simulink model "V_f_control_cinematico_PD"  (R2021b)
settings: Solver=VariableStepAuto  StartTime=0.0  StopTime=110  RelTol=1e-3
libraries: dsparch4 x6, slpidlib x3, simulink x2
settings Model: Creator=bmr  LastModifiedBy=bmr

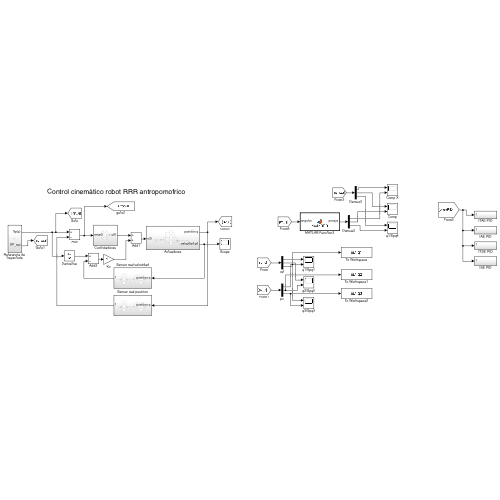
[thumbnail: Simulink's stored preview of the top-level diagram]
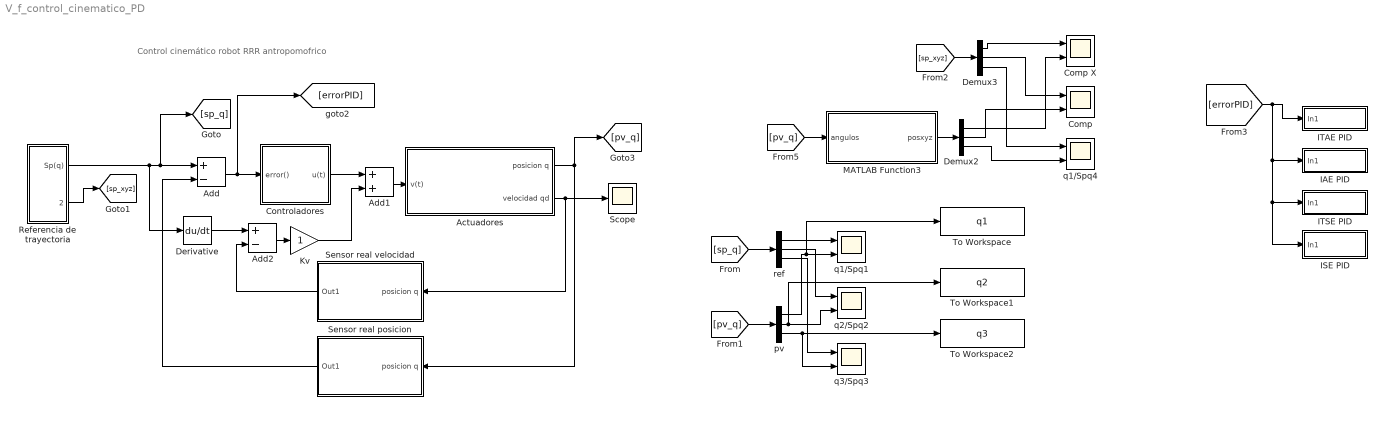
== system V_f_control_cinematico_PD ==
  note: Control cinemático robot RRR antropomofrico
  Actuadores : Subsystem
  Add : Sum  Inputs=+-
  Add1 : Sum
  Add2 : Sum  Inputs=+-
  Comp : Scope  NumInputPorts=2
  Comp X : Scope  NumInputPorts=2
  Controladores : Subsystem
  Demux2 : Demux  Outputs=3
  Demux3 : Demux  Outputs=3
  Derivative : Derivative
  IAE PID : Subsystem
  ISE PID : Subsystem
  ITAE PID : Subsystem
  ITSE PID : Subsystem
  Kv : Gain
  MATLAB Function3 : MATLAB Function  TreatAsAtomicUnit=on
  Referencia de trayectoria : Subsystem
  Scope : Scope
  Sensor real posicion : Subsystem
  Sensor real velocidad : Subsystem
  To Workspace : ToWorkspace  VariableName=q1  SampleTime=0.1
  To Workspace1 : ToWorkspace  VariableName=q2  SampleTime=0.1
  To Workspace2 : ToWorkspace  VariableName=q3  SampleTime=0.1
  pv : Demux  Outputs=3
  q1/Spq1 : Scope  NumInputPorts=2
  q1/Spq4 : Scope  NumInputPorts=2
  q2/Spq2 : Scope  NumInputPorts=2
  q3/Spq3 : Scope  NumInputPorts=2
  ref : Demux  Outputs=3
  wires:
  Add/1 -> [errorPID], Controladores/1(error())
  Actuadores/1(posicion q) -> Sensor real posicion/1(posicion q), [pv_q]
  Actuadores/2(velocidad qd) -> Sensor real velocidad/1(posicion q), Scope/1
  Sensor real posicion/1(Out1) -> Add/2
  [pv_q] -> MATLAB Function3/1(angulos)
  MATLAB Function3/1(posxyz) -> Demux2/1
  Demux2/1 -> Comp X/2
  Demux2/2 -> Comp/2
  Demux2/3 -> q1/Spq4/2
  Referencia de trayectoria/2(SP_xyz) -> [sp_xyz]
  [sp_xyz] -> Demux3/1
  Demux3/1 -> Comp X/1
  Demux3/2 -> Comp/1
  Demux3/3 -> q1/Spq4/1
  Sensor real velocidad/1(Out1) -> Add2/2
  Controladores/1(u(t)) -> Add1/1
  Add1/1 -> Actuadores/1(v(t))
  Derivative/1 -> Add2/1
  Add2/1 -> Kv/1
  Kv/1 -> Add1/2
  ref/1 -> q1/Spq1/1
  pv/1 -> To Workspace/1, q1/Spq1/2
  [pv_q] -> pv/1
  [sp_q] -> ref/1
  ref/2 -> q2/Spq2/1
  pv/2 -> q2/Spq2/2, To Workspace1/1
  pv/3 -> q3/Spq3/2, To Workspace2/1
  ref/3 -> q3/Spq3/1
  [errorPID] -> ISE PID/1(In1), ITSE PID/1(In1), IAE PID/1(In1), ITAE PID/1(In1)
  Referencia de trayectoria/1(Sp(q)) -> [sp_q], Add/1, Derivative/1

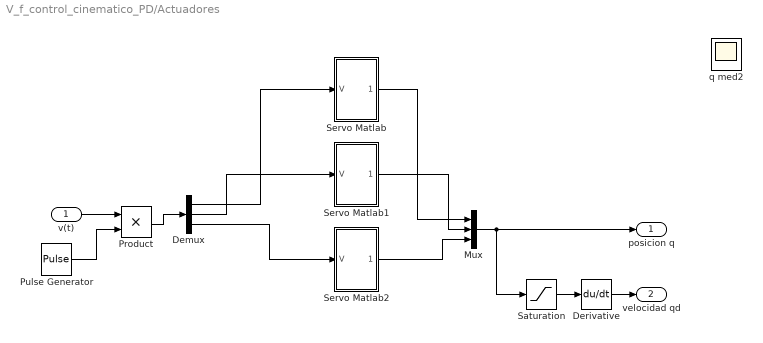
== system V_f_control_cinematico_PD/Actuadores ==
  v(t) : Inport
  Demux : Demux  Outputs=3
  Derivative : Derivative
  Mux : Mux  Inputs=3
  Product : Product
  Pulse Generator : DiscretePulseGenerator  PulseType=Time based  Period=0.001  PulseWidth=50
  Saturation : Saturate  UpperLimit=pi  LowerLimit=-pi
  Servo Matlab : Subsystem
  Servo Matlab1 : Subsystem
  Servo Matlab2 : Subsystem
  q med2 : Scope
  posicion q : Outport
  velocidad qd : Outport  Port=2
  wires:
  Mux/1 -> posicion q/1, Saturation/1
  Derivative/1 -> velocidad qd/1
  Demux/1 -> Servo Matlab/1(V)
  Demux/2 -> Servo Matlab1/1(V)
  Demux/3 -> Servo Matlab2/1(V)
  Servo Matlab2/1(Out1) -> Mux/3
  Servo Matlab1/1(Out1) -> Mux/2
  Servo Matlab/1(Out1) -> Mux/1
  Pulse Generator/1 -> Product/2
  v(t)/1 -> Product/1
  Product/1 -> Demux/1
  Saturation/1 -> Derivative/1

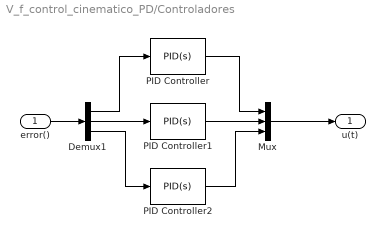
== system V_f_control_cinematico_PD/Controladores ==
  error() : Inport
  Demux1 : Demux  Outputs=3
  Mux : Mux  Inputs=3
  PID Controller : slpidlib/PID Controller  Controller=PID  Form=Parallel  TimeDomain=Continuous-time  UseExternalTs=off  SampleTime=-1  IntegratorMethod=Forward Euler  FilterMethod=Forward Euler  ControllerParametersSource=internal  P=382.208361491745  I=6.52154880893142  D=-1.71522518850909  UseFilter=on  N=222.832759250678  TunerSelectOption=Transfer Function Based (PID Tuner App)  InitialConditionSource=internal  InitialConditionForIntegrator=0  InitialConditionForFilter=0  DifferentiatorICPrevScaledInput=0  ExternalReset=none  TrackingMode=off  Kt=1  LimitOutput=on  SatLimitsSource=internal  UpperSaturationLimit=32000  LowerSaturationLimit=-32000  LinearizeAsGain=on  AntiWindupMode=none  Kb=1  POutMin=[]  POutMax=[]  IOutMin=[]  IOutMax=[]  DOutMin=[]  DOutMax=[]  NOutMin=[]  NOutMax=[]  SumOutMin=[]  SumOutMax=[]  SaturationOutMin=[]  SaturationOutMax=[]  PParamMin=[]  PParamMax=[]  IParamMin=[]  IParamMax=[]  DParamMin=[]  DParamMax=[]  NParamMin=[]  NParamMax=[]  KbParamMin=[]  KbParamMax=[]  KtParamMin=[]  KtParamMax=[]  KbOutMin=[]  KbOutMax=[]  KtOutMin=[]  KtOutMax=[]  IntegratorOutMin=[]  IntegratorOutMax=[]  FilterOutMin=[]  FilterOutMax=[]  SumI1OutMin=[]  SumI1OutMax=[]  SumI2OutMin=[]  SumI2OutMax=[]  SumI3OutMin=[]  SumI3OutMax=[]  SumI4OutMin=[]  SumI4OutMax=[]  SumDOutMin=[]  SumDOutMax=[]  DifferentiatorOutMin=[]  DifferentiatorOutMax=[]  FilterDiffOutCoefMin=[]  FilterDiffOutCoefMax=[]  ReciprocalOutMin=[]  ReciprocalOutMax=[]  SumDenOutMin=[]  SumDenOutMax=[]  SumNumOutMin=[]  SumNumOutMax=[]  DivideOutMin=[]  DivideOutMax=[]  UdiffTsProdOutMin=[]  UdiffTsProdOutMax=[]  NTsProdOutMin=[]  NTsProdOutMax=[]  UintegralTsProdOutMin=[]  UintegralTsProdOutMax=[]  UngainTsProdOutMin=[]  UngainTsProdOutMax=[]  IntegratorContinuousStateAttributes=''  IntegratorStateMustResolveToSignalObject=off  IntegratorRTWStateStorageClass=Auto  FilterContinuousStateAttributes=''  FilterStateMustResolveToSignalObject=off  FilterRTWStateStorageClass=Auto  ParallelPVariant=InternalParameters  IdealPVariant=Disabled  IVariant=InternalParameters  DVariant=InternalParameters  IntegratorVariant=Continuous  SatVariant=Enabled  AWVariant=Passthrough  PCopyVariant=Disabled  TRVariant=Disabled  FdbkBlocksVariant=Forward  IdealPFdbkVariant=Disabled  SatFdbkVariant=Disabled  DerivativeFilterVariant=ContFilter  NVariant=InternalParameters  NCopyVariant=Disabled  FilterICVariant=InternalICsFilter  IntegratorICVariant=InternalICs  ExternalResetVariant=Disabled  TRSumVariant=Passthrough  SumFdbkVariant=Disabled  SumVariant=Sum_PID  TsampFilterVariant=InternalTs  TsampNgainVariant=Passthrough  TsampIntegralVariant=Passthrough  ExternalSaturationOutDataTypeStr=Inherit: Same as second input
  PID Controller1 : slpidlib/PID Controller  Controller=PID  Form=Parallel  TimeDomain=Continuous-time  UseExternalTs=off  SampleTime=-1  IntegratorMethod=Forward Euler  FilterMethod=Forward Euler  ControllerParametersSource=internal  P=380.744284661777  I=6.49105516326343  D=17.2266060618832  UseFilter=on  N=222.832759250678  TunerSelectOption=Transfer Function Based (PID Tuner App)  InitialConditionSource=internal  InitialConditionForIntegrator=0  InitialConditionForFilter=0  DifferentiatorICPrevScaledInput=0  ExternalReset=none  TrackingMode=off  Kt=1  LimitOutput=on  SatLimitsSource=internal  UpperSaturationLimit=32000  LowerSaturationLimit=-32000  LinearizeAsGain=on  AntiWindupMode=none  Kb=1  POutMin=[]  POutMax=[]  IOutMin=[]  IOutMax=[]  DOutMin=[]  DOutMax=[]  NOutMin=[]  NOutMax=[]  SumOutMin=[]  SumOutMax=[]  SaturationOutMin=[]  SaturationOutMax=[]  PParamMin=[]  PParamMax=[]  IParamMin=[]  IParamMax=[]  DParamMin=[]  DParamMax=[]  NParamMin=[]  NParamMax=[]  KbParamMin=[]  KbParamMax=[]  KtParamMin=[]  KtParamMax=[]  KbOutMin=[]  KbOutMax=[]  KtOutMin=[]  KtOutMax=[]  IntegratorOutMin=[]  IntegratorOutMax=[]  FilterOutMin=[]  FilterOutMax=[]  SumI1OutMin=[]  SumI1OutMax=[]  SumI2OutMin=[]  SumI2OutMax=[]  SumI3OutMin=[]  SumI3OutMax=[]  SumI4OutMin=[]  SumI4OutMax=[]  SumDOutMin=[]  SumDOutMax=[]  DifferentiatorOutMin=[]  DifferentiatorOutMax=[]  FilterDiffOutCoefMin=[]  FilterDiffOutCoefMax=[]  ReciprocalOutMin=[]  ReciprocalOutMax=[]  SumDenOutMin=[]  SumDenOutMax=[]  SumNumOutMin=[]  SumNumOutMax=[]  DivideOutMin=[]  DivideOutMax=[]  UdiffTsProdOutMin=[]  UdiffTsProdOutMax=[]  NTsProdOutMin=[]  NTsProdOutMax=[]  UintegralTsProdOutMin=[]  UintegralTsProdOutMax=[]  UngainTsProdOutMin=[]  UngainTsProdOutMax=[]  IntegratorContinuousStateAttributes=''  IntegratorStateMustResolveToSignalObject=off  IntegratorRTWStateStorageClass=Auto  FilterContinuousStateAttributes=''  FilterStateMustResolveToSignalObject=off  FilterRTWStateStorageClass=Auto  ParallelPVariant=InternalParameters  IdealPVariant=Disabled  IVariant=InternalParameters  DVariant=InternalParameters  IntegratorVariant=Continuous  SatVariant=Enabled  AWVariant=Passthrough  PCopyVariant=Disabled  TRVariant=Disabled  FdbkBlocksVariant=Forward  IdealPFdbkVariant=Disabled  SatFdbkVariant=Disabled  DerivativeFilterVariant=ContFilter  NVariant=InternalParameters  NCopyVariant=Disabled  FilterICVariant=InternalICsFilter  IntegratorICVariant=InternalICs  ExternalResetVariant=Disabled  TRSumVariant=Passthrough  SumFdbkVariant=Disabled  SumVariant=Sum_PID  TsampFilterVariant=InternalTs  TsampNgainVariant=Passthrough  TsampIntegralVariant=Passthrough  ExternalSaturationOutDataTypeStr=Inherit: Same as second input
  PID Controller2 : slpidlib/PID Controller  Controller=PID  Form=Parallel  TimeDomain=Continuous-time  UseExternalTs=off  SampleTime=-1  IntegratorMethod=Forward Euler  FilterMethod=Forward Euler  ControllerParametersSource=internal  P=307.461622992245  I=4.77261436567613  D=47.3820560934873  UseFilter=on  N=1.77827193646515  TunerSelectOption=Transfer Function Based (PID Tuner App)  InitialConditionSource=internal  InitialConditionForIntegrator=0  InitialConditionForFilter=0  DifferentiatorICPrevScaledInput=0  ExternalReset=none  TrackingMode=off  Kt=1  LimitOutput=on  SatLimitsSource=internal  UpperSaturationLimit=32000  LowerSaturationLimit=-32000  LinearizeAsGain=on  AntiWindupMode=none  Kb=1  POutMin=[]  POutMax=[]  IOutMin=[]  IOutMax=[]  DOutMin=[]  DOutMax=[]  NOutMin=[]  NOutMax=[]  SumOutMin=[]  SumOutMax=[]  SaturationOutMin=[]  SaturationOutMax=[]  PParamMin=[]  PParamMax=[]  IParamMin=[]  IParamMax=[]  DParamMin=[]  DParamMax=[]  NParamMin=[]  NParamMax=[]  KbParamMin=[]  KbParamMax=[]  KtParamMin=[]  KtParamMax=[]  KbOutMin=[]  KbOutMax=[]  KtOutMin=[]  KtOutMax=[]  IntegratorOutMin=[]  IntegratorOutMax=[]  FilterOutMin=[]  FilterOutMax=[]  SumI1OutMin=[]  SumI1OutMax=[]  SumI2OutMin=[]  SumI2OutMax=[]  SumI3OutMin=[]  SumI3OutMax=[]  SumI4OutMin=[]  SumI4OutMax=[]  SumDOutMin=[]  SumDOutMax=[]  DifferentiatorOutMin=[]  DifferentiatorOutMax=[]  FilterDiffOutCoefMin=[]  FilterDiffOutCoefMax=[]  ReciprocalOutMin=[]  ReciprocalOutMax=[]  SumDenOutMin=[]  SumDenOutMax=[]  SumNumOutMin=[]  SumNumOutMax=[]  DivideOutMin=[]  DivideOutMax=[]  UdiffTsProdOutMin=[]  UdiffTsProdOutMax=[]  NTsProdOutMin=[]  NTsProdOutMax=[]  UintegralTsProdOutMin=[]  UintegralTsProdOutMax=[]  UngainTsProdOutMin=[]  UngainTsProdOutMax=[]  IntegratorContinuousStateAttributes=''  IntegratorStateMustResolveToSignalObject=off  IntegratorRTWStateStorageClass=Auto  FilterContinuousStateAttributes=''  FilterStateMustResolveToSignalObject=off  FilterRTWStateStorageClass=Auto  ParallelPVariant=InternalParameters  IdealPVariant=Disabled  IVariant=InternalParameters  DVariant=InternalParameters  IntegratorVariant=Continuous  SatVariant=Enabled  AWVariant=Passthrough  PCopyVariant=Disabled  TRVariant=Disabled  FdbkBlocksVariant=Forward  IdealPFdbkVariant=Disabled  SatFdbkVariant=Disabled  DerivativeFilterVariant=ContFilter  NVariant=InternalParameters  NCopyVariant=Disabled  FilterICVariant=InternalICsFilter  IntegratorICVariant=InternalICs  ExternalResetVariant=Disabled  TRSumVariant=Passthrough  SumFdbkVariant=Disabled  SumVariant=Sum_PID  TsampFilterVariant=InternalTs  TsampNgainVariant=Passthrough  TsampIntegralVariant=Passthrough  ExternalSaturationOutDataTypeStr=Inherit: Same as second input
  u(t) : Outport
  wires:
  error()/1 -> Demux1/1
  PID Controller2/1 -> Mux/3
  Demux1/1 -> PID Controller/1
  PID Controller1/1 -> Mux/2
  PID Controller/1 -> Mux/1
  Mux/1 -> u(t)/1
  Demux1/2 -> PID Controller1/1
  Demux1/3 -> PID Controller2/1

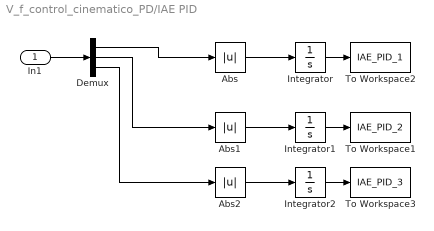
== system V_f_control_cinematico_PD/IAE PID ==
  In1 : Inport
  Abs : Abs
  Abs1 : Abs
  Abs2 : Abs
  Demux : Demux  Outputs=3
  Integrator : Integrator  LimitOutput=on  LowerSaturationLimit=0
  Integrator1 : Integrator  LimitOutput=on  LowerSaturationLimit=0
  Integrator2 : Integrator  LimitOutput=on  LowerSaturationLimit=0
  To Workspace1 : ToWorkspace  VariableName=IAE_PID_2  SampleTime=0.1
  To Workspace2 : ToWorkspace  VariableName=IAE_PID_1  SampleTime=0.1
  To Workspace3 : ToWorkspace  VariableName=IAE_PID_3  SampleTime=0.1
  wires:
  Abs/1 -> Integrator/1
  Integrator/1 -> To Workspace2/1
  Demux/2 -> Abs1/1
  Demux/1 -> Abs/1
  In1/1 -> Demux/1
  Abs1/1 -> Integrator1/1
  Integrator1/1 -> To Workspace1/1
  Integrator2/1 -> To Workspace3/1
  Abs2/1 -> Integrator2/1
  Demux/3 -> Abs2/1

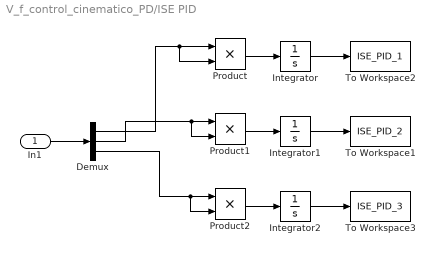
== system V_f_control_cinematico_PD/ISE PID ==
  In1 : Inport
  Demux : Demux  Outputs=3
  Integrator : Integrator  LimitOutput=on  LowerSaturationLimit=0
  Integrator1 : Integrator  LimitOutput=on  LowerSaturationLimit=0
  Integrator2 : Integrator  LimitOutput=on  LowerSaturationLimit=0
  Product : Product
  Product1 : Product
  Product2 : Product
  To Workspace1 : ToWorkspace  VariableName=ISE_PID_2  SampleTime=0.1
  To Workspace2 : ToWorkspace  VariableName=ISE_PID_1  SampleTime=0.1
  To Workspace3 : ToWorkspace  VariableName=ISE_PID_3  SampleTime=0.1
  wires:
  Product/1 -> Integrator/1
  Integrator/1 -> To Workspace2/1
  In1/1 -> Demux/1
  Integrator1/1 -> To Workspace1/1
  Product1/1 -> Integrator1/1
  Product2/1 -> Integrator2/1
  Integrator2/1 -> To Workspace3/1
  Demux/1 -> Product/2, Product/1
  Demux/2 -> Product1/2, Product1/1
  Demux/3 -> Product2/2, Product2/1

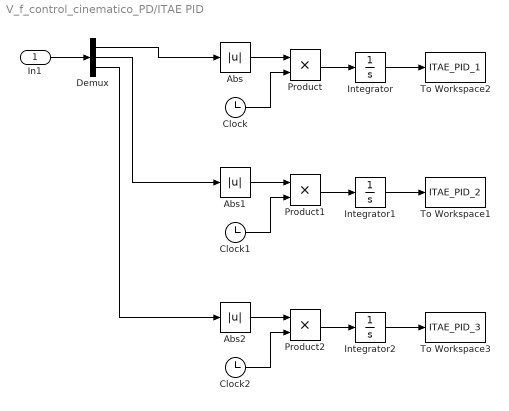
== system V_f_control_cinematico_PD/ITAE PID ==
  In1 : Inport
  Abs : Abs
  Abs1 : Abs
  Abs2 : Abs
  Clock : Clock
  Clock1 : Clock
  Clock2 : Clock
  Demux : Demux  Outputs=3
  Integrator : Integrator  LimitOutput=on  LowerSaturationLimit=0
  Integrator1 : Integrator  LimitOutput=on  LowerSaturationLimit=0
  Integrator2 : Integrator  LimitOutput=on  LowerSaturationLimit=0
  Product : Product
  Product1 : Product
  Product2 : Product
  To Workspace1 : ToWorkspace  VariableName=ITAE_PID_2  SampleTime=0.1
  To Workspace2 : ToWorkspace  VariableName=ITAE_PID_1  SampleTime=0.1
  To Workspace3 : ToWorkspace  VariableName=ITAE_PID_3  SampleTime=0.1
  wires:
  Clock/1 -> Product/2
  Abs/1 -> Product/1
  Integrator/1 -> To Workspace2/1
  Product/1 -> Integrator/1
  Clock1/1 -> Product1/2
  Product1/1 -> Integrator1/1
  Abs1/1 -> Product1/1
  Integrator1/1 -> To Workspace1/1
  Clock2/1 -> Product2/2
  Product2/1 -> Integrator2/1
  Abs2/1 -> Product2/1
  Integrator2/1 -> To Workspace3/1
  In1/1 -> Demux/1
  Demux/1 -> Abs/1
  Demux/2 -> Abs1/1
  Demux/3 -> Abs2/1

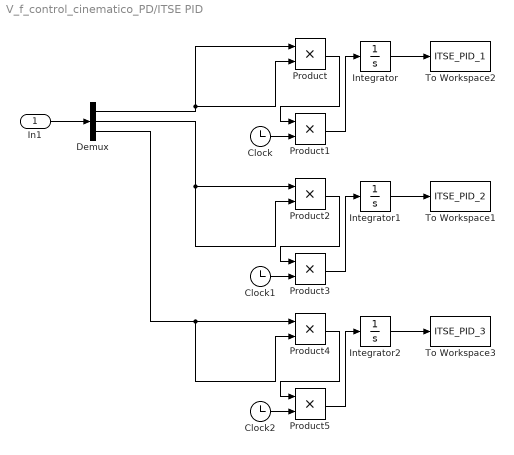
== system V_f_control_cinematico_PD/ITSE PID ==
  In1 : Inport
  Clock : Clock
  Clock1 : Clock
  Clock2 : Clock
  Demux : Demux  Outputs=3
  Integrator : Integrator  LimitOutput=on  LowerSaturationLimit=0
  Integrator1 : Integrator  LimitOutput=on  LowerSaturationLimit=0
  Integrator2 : Integrator  LimitOutput=on  LowerSaturationLimit=0
  Product{,1..5} (6 alike) : Product
  To Workspace1 : ToWorkspace  VariableName=ITSE_PID_2  SampleTime=0.1
  To Workspace2 : ToWorkspace  VariableName=ITSE_PID_1  SampleTime=0.1
  To Workspace3 : ToWorkspace  VariableName=ITSE_PID_3  SampleTime=0.1
  wires:
  Demux/1 -> Product/1, Product/2
  Integrator/1 -> To Workspace2/1
  Product/1 -> Product1/1
  Clock/1 -> Product1/2
  Product1/1 -> Integrator/1
  In1/1 -> Demux/1
  Integrator1/1 -> To Workspace1/1
  Product2/1 -> Product3/1
  Product3/1 -> Integrator1/1
  Demux/2 -> Product2/2, Product2/1
  Clock1/1 -> Product3/2
  Product4/1 -> Product5/1
  Product5/1 -> Integrator2/1
  Clock2/1 -> Product5/2
  Demux/3 -> Product4/2, Product4/1
  Integrator2/1 -> To Workspace3/1

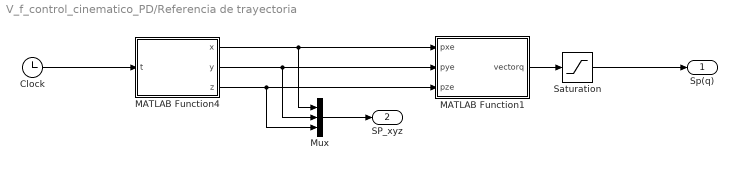
== system V_f_control_cinematico_PD/Referencia de trayectoria ==
  Clock : Clock
  MATLAB Function1 : MATLAB Function  TreatAsAtomicUnit=on
  MATLAB Function4 : MATLAB Function  TreatAsAtomicUnit=on
  Mux : Mux  Inputs=3
  Saturation : Saturate  UpperLimit=1.57  LowerLimit=-1.57
  Sp(q) : Outport
  SP_xyz : Outport  Port=2
  wires:
  MATLAB Function1/1(vectorq) -> Saturation/1
  Clock/1 -> MATLAB Function4/1(t)
  MATLAB Function4/3(z) -> Mux/3, MATLAB Function1/3(pze)
  MATLAB Function4/2(y) -> Mux/2, MATLAB Function1/2(pye)
  MATLAB Function4/1(x) -> Mux/1, MATLAB Function1/1(pxe)
  Saturation/1 -> Sp(q)/1
  Mux/1 -> SP_xyz/1

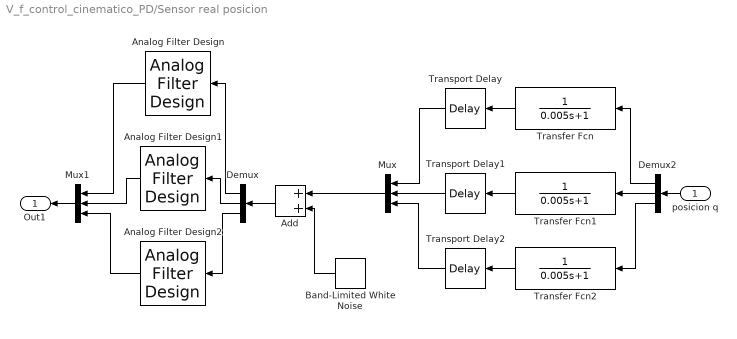
== system V_f_control_cinematico_PD/Sensor real posicion ==
  posicion q : Inport
  Add : Sum
  Analog Filter Design : dsparch4/Analog Filter Design  method=Butterworth  filttype=Lowpass  N=8  Wlo=30  Whi=80  Rp=2  Rs=40
  Analog Filter Design1 : dsparch4/Analog Filter Design  method=Butterworth  filttype=Lowpass  N=8  Wlo=30  Whi=80  Rp=2  Rs=40
  Analog Filter Design2 : dsparch4/Analog Filter Design  method=Butterworth  filttype=Lowpass  N=8  Wlo=30  Whi=80  Rp=2  Rs=40
  Band-Limited White Noise : simulink/Sources/Band-Limited White Noise  Cov=[0.001]  Ts=0.1  seed=[23341]
  Demux : Demux  Outputs=3
  Demux2 : Demux  Outputs=3
  Mux : Mux  Inputs=3
  Mux1 : Mux  Inputs=3
  Transfer Fcn : TransferFcn  Denominator=[0.005 1]
  Transfer Fcn1 : TransferFcn  Denominator=[0.005 1]
  Transfer Fcn2 : TransferFcn  Denominator=[0.005 1]
  Transport Delay : TransportDelay  DelayTime=0.05
  Transport Delay1 : TransportDelay  DelayTime=0.05
  Transport Delay2 : TransportDelay  DelayTime=0.05
  Out1 : Outport
  wires:
  Transfer Fcn1/1 -> Transport Delay1/1
  Demux2/3 -> Transfer Fcn2/1
  Transfer Fcn/1 -> Transport Delay/1
  Demux2/2 -> Transfer Fcn1/1
  Transport Delay/1 -> Mux/1
  Transfer Fcn2/1 -> Transport Delay2/1
  Transport Delay1/1 -> Mux/2
  Transport Delay2/1 -> Mux/3
  Demux2/1 -> Transfer Fcn/1
  posicion q/1 -> Demux2/1
  Band-Limited White Noise/1 -> Add/2
  Mux/1 -> Add/1
  Add/1 -> Demux/1
  Demux/1 -> Analog Filter Design/1
  Demux/2 -> Analog Filter Design1/1
  Demux/3 -> Analog Filter Design2/1
  Mux1/1 -> Out1/1
  Analog Filter Design/1 -> Mux1/1
  Analog Filter Design1/1 -> Mux1/2
  Analog Filter Design2/1 -> Mux1/3

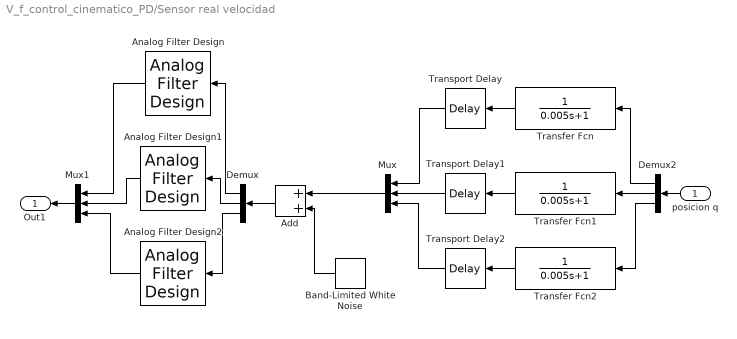
== system V_f_control_cinematico_PD/Sensor real velocidad ==
  posicion q : Inport
  Add : Sum
  Analog Filter Design : dsparch4/Analog Filter Design  method=Butterworth  filttype=Lowpass  N=8  Wlo=30  Whi=80  Rp=2  Rs=40
  Analog Filter Design1 : dsparch4/Analog Filter Design  method=Butterworth  filttype=Lowpass  N=8  Wlo=30  Whi=80  Rp=2  Rs=40
  Analog Filter Design2 : dsparch4/Analog Filter Design  method=Butterworth  filttype=Lowpass  N=8  Wlo=30  Whi=80  Rp=2  Rs=40
  Band-Limited White Noise : simulink/Sources/Band-Limited White Noise  Cov=[0.001]  Ts=0.1  seed=[23341]
  Demux : Demux  Outputs=3
  Demux2 : Demux  Outputs=3
  Mux : Mux  Inputs=3
  Mux1 : Mux  Inputs=3
  Transfer Fcn : TransferFcn  Denominator=[0.005 1]
  Transfer Fcn1 : TransferFcn  Denominator=[0.005 1]
  Transfer Fcn2 : TransferFcn  Denominator=[0.005 1]
  Transport Delay : TransportDelay  DelayTime=0.05
  Transport Delay1 : TransportDelay  DelayTime=0.05
  Transport Delay2 : TransportDelay  DelayTime=0.05
  Out1 : Outport
  wires:
  Transfer Fcn1/1 -> Transport Delay1/1
  Demux2/3 -> Transfer Fcn2/1
  Transfer Fcn/1 -> Transport Delay/1
  Demux2/2 -> Transfer Fcn1/1
  Transport Delay/1 -> Mux/1
  Transfer Fcn2/1 -> Transport Delay2/1
  Transport Delay1/1 -> Mux/2
  Transport Delay2/1 -> Mux/3
  Demux2/1 -> Transfer Fcn/1
  posicion q/1 -> Demux2/1
  Band-Limited White Noise/1 -> Add/2
  Mux/1 -> Add/1
  Add/1 -> Demux/1
  Demux/1 -> Analog Filter Design/1
  Demux/2 -> Analog Filter Design1/1
  Demux/3 -> Analog Filter Design2/1
  Mux1/1 -> Out1/1
  Analog Filter Design/1 -> Mux1/1
  Analog Filter Design1/1 -> Mux1/2
  Analog Filter Design2/1 -> Mux1/3

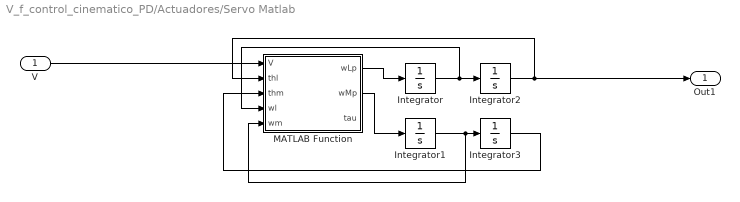
== system V_f_control_cinematico_PD/Actuadores/Servo Matlab ==
  V : Inport
  Integrator : Integrator  UpperSaturationLimit=pi/2  LowerSaturationLimit=-pi/2
  Integrator1 : Integrator
  Integrator2 : Integrator  LimitOutput=on  UpperSaturationLimit=pi/2  LowerSaturationLimit=-pi/2
  Integrator3 : Integrator  UpperSaturationLimit=pi/2  LowerSaturationLimit=-pi/2
  MATLAB Function : MATLAB Function  TreatAsAtomicUnit=on
  Out1 : Outport
  wires:
  V/1 -> MATLAB Function/1(V)
  Integrator2/1 -> Out1/1, MATLAB Function/2(thl)
  Integrator/1 -> Integrator2/1, MATLAB Function/4(wl)
  MATLAB Function/1(wLp) -> Integrator/1
  Integrator3/1 -> MATLAB Function/3(thm)
  MATLAB Function/2(wMp) -> Integrator1/1
  Integrator1/1 -> Integrator3/1, MATLAB Function/5(wm)

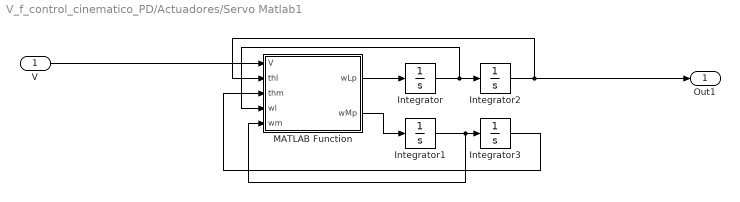
== system V_f_control_cinematico_PD/Actuadores/Servo Matlab1 ==
  V : Inport
  Integrator : Integrator  UpperSaturationLimit=pi/2  LowerSaturationLimit=-pi/2
  Integrator1 : Integrator
  Integrator2 : Integrator  InitialCondition=pi/2  LimitOutput=on  UpperSaturationLimit=pi/2  LowerSaturationLimit=-pi/2
  Integrator3 : Integrator  UpperSaturationLimit=pi/2  LowerSaturationLimit=-pi/2
  MATLAB Function : MATLAB Function  TreatAsAtomicUnit=on
  Out1 : Outport
  wires:
  V/1 -> MATLAB Function/1(V)
  Integrator2/1 -> Out1/1, MATLAB Function/2(thl)
  Integrator/1 -> Integrator2/1, MATLAB Function/4(wl)
  MATLAB Function/1(wLp) -> Integrator/1
  Integrator3/1 -> MATLAB Function/3(thm)
  MATLAB Function/2(wMp) -> Integrator1/1
  Integrator1/1 -> Integrator3/1, MATLAB Function/5(wm)

== system V_f_control_cinematico_PD/Actuadores/Servo Matlab2 ==
  V : Inport
  Integrator : Integrator  InitialCondition=-pi/2  UpperSaturationLimit=pi/2  LowerSaturationLimit=-pi/2
  Integrator1 : Integrator
  Integrator2 : Integrator  LimitOutput=on  UpperSaturationLimit=pi/2  LowerSaturationLimit=-pi/2
  Integrator3 : Integrator  UpperSaturationLimit=pi/2  LowerSaturationLimit=-pi/2
  MATLAB Function : MATLAB Function  TreatAsAtomicUnit=on
  Out1 : Outport
  wires:
  V/1 -> MATLAB Function/1(V)
  Integrator2/1 -> Out1/1, MATLAB Function/2(thl)
  Integrator/1 -> Integrator2/1, MATLAB Function/4(wl)
  MATLAB Function/1(wLp) -> Integrator/1
  Integrator3/1 -> MATLAB Function/3(thm)
  MATLAB Function/2(wMp) -> Integrator1/1
  Integrator1/1 -> Integrator3/1, MATLAB Function/5(wm)

== matlab function V_f_control_cinematico_PD/Actuadores/Servo Matlab/MATLAB Function ==
  data: V input; wLp output; thl input; thm input; wl input; wm input; wMp output; tau output
function [wLp,wMp,tau] = servomotor(V, thl,thm, wl, wm)
Kt = 1280.2;  % Torsional rigidity
Km = 10;      % Motor constant
Jm = 0.5;     % Motor inertia
Jl = 50*Jm;   % Load inertia
N = 20;       % Gear ratio
Bm = 0.1;     % Rotor viscous friction
Bl = 25;      % Load viscous friction
R = 20;       % Armature resistance
wLp = (-(Kt/Jl)*(thl - (thm/N))) - ((Bl*wl)/Jl);
wMp = (Km/Jm) * ((V - Km * wm)/R) - ((Bm * wm)/Jm) + (Kt/(N*Jm))*(thl - (thm/N));
%% https://www.mathworks.com/help/mpc/ug/servomechanism-controller.html?searchHighlight=mpc%20dc%20motor&s_tid=doc_srchtitle %%
% Torque maquina
tau = (Kt * thl) -((Kt/N)*thm);

== matlab function V_f_control_cinematico_PD/Referencia de trayectoria/MATLAB Function1 ==
  data: pxe input size=1; vectorq output size=3; pye input size=1; pze input size=1
function vectorq = cininvRRR(pxe,pye,pze)
%% Valores 
L1=0.2;L2=0.2;L3=0.2;
%% angulos
q1=atan2(pye,pxe);
cq3=(pxe^2 +pye^2 +pze^2 -L2^2 -L3^2)/(2*L2*L3);
%% Condicionante para la variable cq3
if (cq3>=1)
    cq3=1;
else
    cq3=0.001;
end 

q3=atan2(sqrt(1-cq3),cq3);
beta=atan2(pze,sqrt(pxe^2 +pye^2));
alfa=atan2(L3*sin(q3),L2 +L3*cq3);
q2=beta-alfa;
vectorq=[q1;q2;q3];

== matlab function V_f_control_cinematico_PD/MATLAB Function3 ==
  data: angulos input size=3; posxyz output size=3
%% Funcion cinematica directa
function posxyz = cindinRRR(angulos)
%% Vector angulo de 3 dim.
th1=angulos(1);
th2=angulos(2);
th3=angulos(3);
%% Valores eslabones
L1=0.2;L2=0.2;L3=0.2;
%% pos
xe=cos(th1)*(L3*cos(th2+th3) + L2*cos(th2));
ye=sin(th1)*(L3*cos(th2+th3) + L2*cos(th2));
ze=L1+(L3*sin(th2+th3)) +L2*sin(th2);
posxyz=[xe;ye;ze];

== matlab function V_f_control_cinematico_PD/Referencia de trayectoria/MATLAB Function4 ==
  data: x output; t input; y output; z output
function [x,y,z] = Trayectoria(t)

if (t>=0) && (t<15)
    x = 0.2;
    y = 0.0;
    z = 0.4;

elseif (t>=15) && (t<30) 
    x = 0.2;
    y = 0.0;
    z = 0.0;
elseif (t>=30) && (t<45)
    x = 0.0;
    y = 0.2;
    z = 0.0;

elseif (t>=45) && (t<60)
    x = 0.2;
    y = 0.0;
    z = 0.0;

elseif (t>=60) && (t<75)
    x = 0.0;
    y = -0.2;
    z = 0.0;


elseif (t>=75) && (t<90)
    x = 0.4;
    y = 0.0;
    z = 0.2;


elseif (t>=90) && (t<105)
    x = 0.0;
    y = -0.4;
    z = 0.2;

else
    x = 0.4;
    y = 0.0;
    z = 0.2;
end

== matlab function V_f_control_cinematico_PD/Actuadores/Servo Matlab1/MATLAB Function ==
  data: V input; wLp output; thl input; thm input; wl input; wm input; wMp output
function [wLp,wMp] = servomotor(V, thl,thm, wl, wm)
Kt = 1280.2;  % Torsional rigidity
Km = 10;      % Motor constant
Jm = 0.5;     % Motor inertia
Jl = 50*Jm;   % Load inertia
N = 20;       % Gear ratio
Bm = 0.1;     % Rotor viscous friction
Bl = 25;      % Load viscous friction
R = 20;       % Armature resistance
wLp = (-(Kt/Jl)*(thl - (thm/N))) - ((Bl*wl)/Jl);
wMp = (Km/Jm) * ((V - Km * wm)/R) - ((Bm * wm)/Jm) + (Kt/(N*Jm))*(thl - (thm/N));
%% https://www.mathworks.com/help/mpc/ug/servomechanism-controller.html?searchHighlight=mpc%20dc%20motor&s_tid=doc_srchtitle %%

== matlab function V_f_control_cinematico_PD/Actuadores/Servo Matlab2/MATLAB Function ==
  data: V input; wLp output; thl input; thm input; wl input; wm input; wMp output
function [wLp,wMp] = servomotor(V, thl,thm, wl, wm)
Kt = 1280.2;  % Torsional rigidity
Km = 10;      % Motor constant
Jm = 0.5;     % Motor inertia
Jl = 50*Jm;   % Load inertia
N = 20;       % Gear ratio
Bm = 0.1;     % Rotor viscous friction
Bl = 25;      % Load viscous friction
R = 20;       % Armature resistance
wLp = (-(Kt/Jl)*(thl - (thm/N))) - ((Bl*wl)/Jl);
wMp = (Km/Jm) * ((V - Km * wm)/R) - ((Bm * wm)/Jm) + (Kt/(N*Jm))*(thl - (thm/N));
%% https://www.mathworks.com/help/mpc/ug/servomechanism-controller.html?searchHighlight=mpc%20dc%20motor&s_tid=doc_srchtitle %%
